simulink model "gm_IP_Core_SS_Switch_and_PWM"  (R2023a)
settings: Solver=VariableStepAuto  StartTime=0.0  StopTime=0.0004  RelTol=1e-3
undefined symbols (not defined in the file or in its folder): f_FPGA_clk, T_FPGA_clk
libraries: hdlsllib x9, simulink x2
(part 3 of 3)

== system gm_IP_Core_SS_Switch_and_PWM/PWM_and_Switching_Signal_Control1/GenPWM/Triangle shift2 ==
  note: Shifts triangle_in signal, if:
      | -direction of triangle_in is down
      | -user input demands a shift smaller than 1/2 of the period
  note: Shifts triangle_in signal, if:
      | -direction of triangle_in is up
      | -user input demands a shift smaller than 1/2 of the period
  note: Shifts triangle_in signal, if:
      | -direction of triangle_in is up
      | -user input demands a shift larger than 1/2 of the period
  note: Shifts triangle_in signal, if:
      | -direction of triangle_in is down
      | -user input demands a shift larger than 1/2 of the period
  note: Detects, if the triangle_wave is increasing or decreasing
  note: modifies triangle_in signal,
      | if the user demands a shift larger than 1/2 period
  triangle_in : Inport
  triangle_shift : Inport  Port=2
  0 : Constant  Value=0  OutDataTypeStr=boolean  SampleTime=T_FPGA_clk
  Data Type Conversion : DataTypeConversion  OutDataTypeStr=fixdt(1,19,17)  SaturateOnIntegerOverflow=off  RndMeth=Floor
  Data Type Conversion1 : DataTypeConversion  OutDataTypeStr=fixdt(1,20,17)  SaturateOnIntegerOverflow=off  RndMeth=Floor
  Delay1 : Delay  DelayLength=1
  Delay2 : Delay  DelayLength=1
  Gain : Gain  Gain=2  OutDataTypeStr=fixdt(1,20,17)
  Gain1 : Gain  Gain=2  OutDataTypeStr=fixdt(1,20,17)
  Relational Operator1 : RelationalOperator  Operator=<=  OutDataTypeStr=boolean  InputSameDT=off
  Relational Operator7 : RelationalOperator  OutDataTypeStr=boolean  InputSameDT=off
  Subsystem : Subsystem
  Subsystem1 : Subsystem
  Subsystem2 : Subsystem
  Subsystem3 : Subsystem
  Sum10 : Sum  Inputs=|-+  OutDataTypeStr=fixdt(1,20,17)
  or : Switch  Criteria=u2 > Threshold  SaturateOnIntegerOverflow=off  InputSameDT=off
  standardized peak of triangle : Constant  OutDataTypeStr=fixdt(0,21,17)  SampleTime=T_FPGA_clk
  sw1 : Switch  Criteria=u2 > Threshold  OutDataTypeStr=fixdt(1,18,16)  SaturateOnIntegerOverflow=off  InputSameDT=off
  sw2 : Switch  Criteria=u2 > Threshold  SaturateOnIntegerOverflow=off  InputSameDT=off
  sw3 : Switch  Criteria=u2 > Threshold  SaturateOnIntegerOverflow=off  InputSameDT=off
  sw4 : Switch  Criteria=u2 > Threshold  Threshold=1  OutDataTypeStr=fixdt(1,20,17)  SaturateOnIntegerOverflow=off  InputSameDT=off
  triangle_sig : Outport  VectorParamsAs1DForOutWhenUnconnected=off
  wires:
  Subsystem3/1(shifted triangle_in signal) -> sw2/3
  Subsystem2/2(enable_out) -> sw1/2
  Subsystem2/1(shifted triangle_in signal) -> sw1/1
  Subsystem1/1(shifted triangle_in signal) -> sw3/1
  Subsystem1/2(enable_out) -> sw3/2, or/1, or/2
  Subsystem/2(enable_out) -> or/3
  Subsystem/1(shifted triangle_in signal) -> sw3/3
  0/1 -> Subsystem/1(Zero_input), Subsystem1/5(Zero_input), Subsystem2/4(Zero_input)
  Delay1/1 -> Relational Operator1/2
  Relational Operator1/1 -> Subsystem2/5(direction down), Subsystem/5(direction down)  "direction down"
  triangle_in/1 -> Data Type Conversion1/1
  Data Type Conversion/1 -> Gain/1
  sw2/1 -> sw1/3
  Gain1/1 -> Sum10/1
  triangle_shift/1 -> Data Type Conversion/1
  standardized peak of triangle/1 -> Gain1/1, Subsystem1/1(standardized peak of triangle), Subsystem2/3(standardized peak of triangle)  "standardized peak of triangle"
  sw1/1 -> triangle_sig/1
  Sum10/1 -> sw4/1
  Gain/1 -> sw4/2, sw4/3, Subsystem1/3(converted triangle_shift), Subsystem/2(converted triangle_shift), Sum10/2  "converted triangle_shift"
  sw4/1 -> Subsystem2/2(modified triangle_shift), Subsystem1/4(modified triangle_shift), Subsystem/3(modified triangle_shift), Subsystem3/2(modified triangle_shift)  "modified triangle_shift"
  or/1 -> sw2/2
  Relational Operator7/1 -> Subsystem3/3(direction up), Subsystem1/6(direction up)  "direction up"
  sw3/1 -> sw2/1
  Data Type Conversion1/1 -> Relational Operator7/1, Delay2/1, Delay1/1, Relational Operator1/1, Subsystem1/2(triangle_in), Subsystem/4(triangle_in), Subsystem2/1(triangle_in), Subsystem3/1(triangle_in)  "triangle_in"
  Delay2/1 -> Relational Operator7/2

== system gm_IP_Core_SS_Switch_and_PWM/PWM_and_Switching_Signal_Control/GenPWM/Counter Ctrl/Delay6_controlled ==
  in0 : Inport  OutDataTypeStr=boolean  SampleTime=1e-08
  stateControl : EnablePort  OutDataTypeStr=boolean
  Delay6 : Delay  DelayLength=double(1)  InitialCondition=0  SampleTime=1e-08
  out0 : Outport  OutDataTypeStr=boolean  SampleTime=1e-08
  wires:
  Delay6/1 -> out0/1
  in0/1 -> Delay6/1

== system gm_IP_Core_SS_Switch_and_PWM/PWM_and_Switching_Signal_Control/GenPWM/Counter Ctrl/Delay_controlled ==
  in0 : Inport  OutDataTypeStr=fixdt(0, 25, 26)  SampleTime=1e-08
  stateControl : EnablePort  OutDataTypeStr=boolean
  Delay : Delay  DelayLength=double(1)  InitialCondition=0  SampleTime=1e-08
  out0 : Outport  OutDataTypeStr=fixdt(0, 25, 26)  SampleTime=1e-08
  wires:
  Delay/1 -> out0/1
  in0/1 -> Delay/1

== system gm_IP_Core_SS_Switch_and_PWM/PWM_and_Switching_Signal_Control/GenPWM/Triangle shift/Subsystem ==
  Zero_input : Inport  OutDataTypeStr=boolean  PortDimensions=1  SampleTime=1e-08
  converted triangle_shift : Inport  Port=2  OutDataTypeStr=fixdt(1, 20, 17)  PortDimensions=1  SampleTime=1e-08
  modified triangle_shift : Inport  Port=3  OutDataTypeStr=fixdt(1, 20, 17)  PortDimensions=1  SampleTime=1e-08
  triangle_in : Inport  Port=4  OutDataTypeStr=fixdt(1, 20, 17)  PortDimensions=1  SampleTime=1e-08
  direction down : Inport  Port=5  OutDataTypeStr=boolean  PortDimensions=1  SampleTime=1e-08
  Relational Operator11 : RelationalOperator  Operator=<=  OutDataTypeStr=boolean  SampleTime=1e-08  InputSameDT=off
  Sum8 : Sum  Inputs=+-  AccumDataTypeStr=fixdt(1, 21, 17)  OutDataTypeStr=fixdt(1, 21, 17)  SampleTime=1e-08
  Unary Minus : UnaryMinus  SampleTime=1e-08
  and2_1 : Switch  Criteria=u2 > Threshold  Threshold=double(0)  OutDataTypeStr=boolean  SampleTime=1e-08  SaturateOnIntegerOverflow=off  InputSameDT=off
  and2_2 : Switch  Criteria=u2 > Threshold  Threshold=double(0)  OutDataTypeStr=boolean  SampleTime=1e-08  SaturateOnIntegerOverflow=off  InputSameDT=off
  shifted triangle_in signal : Outport  SampleTime=1e-08
  enable_out : Outport  Port=2  SampleTime=1e-08
  wires:
  Relational Operator11/1 -> and2_1/2
  Sum8/1 -> shifted triangle_in signal/1
  Unary Minus/1 -> Sum8/1, Relational Operator11/2
  and2_1/1 -> and2_2/1
  and2_2/1 -> enable_out/1
  Zero_input/1 -> and2_2/3, and2_1/3
  converted triangle_shift/1 -> and2_1/1
  modified triangle_shift/1 -> Unary Minus/1
  triangle_in/1 -> Sum8/2, Relational Operator11/1
  direction down/1 -> and2_2/2

== system gm_IP_Core_SS_Switch_and_PWM/PWM_and_Switching_Signal_Control/GenPWM/Triangle shift/Subsystem1 ==
  standardized peak of triangle : Inport  OutDataTypeStr=fixdt(0, 21, 17)  PortDimensions=1  SampleTime=1e-08
  triangle_in : Inport  Port=2  OutDataTypeStr=fixdt(1, 20, 17)  PortDimensions=1  SampleTime=1e-08
  converted triangle_shift : Inport  Port=3  OutDataTypeStr=fixdt(1, 20, 17)  PortDimensions=1  SampleTime=1e-08
  modified triangle_shift : Inport  Port=4  OutDataTypeStr=fixdt(1, 20, 17)  PortDimensions=1  SampleTime=1e-08
  Zero_input : Inport  Port=5  OutDataTypeStr=boolean  PortDimensions=1  SampleTime=1e-08
  direction up : Inport  Port=6  OutDataTypeStr=boolean  PortDimensions=1  SampleTime=1e-08
  Relational Operator2 : RelationalOperator  OutDataTypeStr=boolean  SampleTime=1e-08  InputSameDT=off
  Sum11_stage2 : Sum  AccumDataTypeStr=fixdt(1, 24, 17)  OutDataTypeStr=fixdt(1, 24, 17)  SampleTime=1e-08
  Sum11_stage3 : Sum  Inputs=+-  AccumDataTypeStr=fixdt(1, 24, 17)  OutDataTypeStr=fixdt(1, 21, 17)  SampleTime=1e-08
  Sum6 : Sum  AccumDataTypeStr=fixdt(1, 23, 17)  OutDataTypeStr=fixdt(1, 23, 17)  SampleTime=1e-08
  and1_1 : Switch  Criteria=u2 > Threshold  Threshold=double(0)  OutDataTypeStr=boolean  SampleTime=1e-08  SaturateOnIntegerOverflow=off  InputSameDT=off
  and1_2 : Switch  Criteria=u2 > Threshold  Threshold=double(0)  OutDataTypeStr=boolean  SampleTime=1e-08  SaturateOnIntegerOverflow=off  InputSameDT=off
  shifted triangle_in signal : Outport  SampleTime=1e-08
  enable_out : Outport  Port=2  SampleTime=1e-08
  wires:
  Relational Operator2/1 -> and1_1/2
  Sum11_stage3/1 -> shifted triangle_in signal/1
  Sum6/1 -> Sum11_stage2/2, Relational Operator2/2
  and1_1/1 -> and1_2/1
  and1_2/1 -> enable_out/1
  Sum11_stage2/1 -> Sum11_stage3/1
  standardized peak of triangle/1 -> Sum6/2, Sum11_stage2/1
  triangle_in/1 -> Sum11_stage3/2, Relational Operator2/1
  converted triangle_shift/1 -> and1_1/1
  modified triangle_shift/1 -> Sum6/1
  Zero_input/1 -> and1_2/3, and1_1/3
  direction up/1 -> and1_2/2

== system gm_IP_Core_SS_Switch_and_PWM/PWM_and_Switching_Signal_Control/GenPWM/Triangle shift/Subsystem2 ==
  triangle_in : Inport  OutDataTypeStr=fixdt(1, 20, 17)  PortDimensions=1  SampleTime=1e-08
  modified triangle_shift : Inport  Port=2  OutDataTypeStr=fixdt(1, 20, 17)  PortDimensions=1  SampleTime=1e-08
  standardized peak of triangle : Inport  Port=3  OutDataTypeStr=fixdt(0, 21, 17)  PortDimensions=1  SampleTime=1e-08
  Zero_input : Inport  Port=4  OutDataTypeStr=boolean  PortDimensions=1  SampleTime=1e-08
  direction down : Inport  Port=5  OutDataTypeStr=boolean  PortDimensions=1  SampleTime=1e-08
  Relational Operator9 : RelationalOperator  OutDataTypeStr=boolean  SampleTime=1e-08  InputSameDT=off
  Sum1 : Sum  Inputs=+-  AccumDataTypeStr=fixdt(1, 23, 17)  OutDataTypeStr=fixdt(1, 23, 17)  SampleTime=1e-08
  Sum5_stage2 : Sum  AccumDataTypeStr=fixdt(1, 24, 17)  OutDataTypeStr=fixdt(1, 24, 17)  SampleTime=1e-08
  Sum5_stage3 : Sum  Inputs=+-  AccumDataTypeStr=fixdt(1, 24, 17)  OutDataTypeStr=fixdt(1, 21, 17)  SampleTime=1e-08
  and : Switch  Criteria=u2 > Threshold  Threshold=double(0)  OutDataTypeStr=boolean  SampleTime=1e-08  SaturateOnIntegerOverflow=off  InputSameDT=off
  shifted triangle_in signal : Outport  SampleTime=1e-08
  enable_out : Outport  Port=2  SampleTime=1e-08
  wires:
  Relational Operator9/1 -> and/1
  Sum1/1 -> Sum5_stage2/1, Relational Operator9/2
  Sum5_stage3/1 -> shifted triangle_in signal/1
  and/1 -> enable_out/1
  Sum5_stage2/1 -> Sum5_stage3/1
  triangle_in/1 -> Sum5_stage3/2, Relational Operator9/1
  modified triangle_shift/1 -> Sum1/2
  standardized peak of triangle/1 -> Sum5_stage2/2, Sum1/1
  Zero_input/1 -> and/3
  direction down/1 -> and/2

== system gm_IP_Core_SS_Switch_and_PWM/PWM_and_Switching_Signal_Control/GenPWM/Triangle shift/Subsystem3 ==
  triangle_in : Inport  OutDataTypeStr=fixdt(1, 20, 17)  PortDimensions=1  SampleTime=1e-08
  modified triangle_shift : Inport  Port=2  OutDataTypeStr=fixdt(1, 20, 17)  PortDimensions=1  SampleTime=1e-08
  direction up : Inport  Port=3  OutDataTypeStr=boolean  PortDimensions=1  SampleTime=1e-08
  Relational Operator6 : RelationalOperator  Operator=<=  OutDataTypeStr=boolean  SampleTime=1e-08  InputSameDT=off
  Sum2 : Sum  Inputs=+-  AccumDataTypeStr=fixdt(1, 21, 17)  OutDataTypeStr=fixdt(1, 21, 17)  SampleTime=1e-08
  Sum3 : Sum  Inputs=+-  AccumDataTypeStr=fixdt(1, 21, 17)  OutDataTypeStr=fixdt(1, 21, 17)  SampleTime=1e-08
  Sum4 : Sum  AccumDataTypeStr=fixdt(1, 21, 17)  OutDataTypeStr=fixdt(1, 21, 17)  SampleTime=1e-08
  Switch3 : Switch  Criteria=u2 > Threshold  Threshold=double(0)  OutDataTypeStr=fixdt(1, 21, 17)  SampleTime=1e-08  SaturateOnIntegerOverflow=off  InputSameDT=off
  sw : Switch  Criteria=u2 > Threshold  Threshold=double(0)  OutDataTypeStr=fixdt(1, 21, 17)  SampleTime=1e-08  SaturateOnIntegerOverflow=off  InputSameDT=off
  shifted triangle_in signal : Outport  SampleTime=1e-08
  wires:
  Relational Operator6/1 -> Switch3/2
  Sum2/1 -> Switch3/1
  Sum3/1 -> Switch3/3
  Sum4/1 -> sw/3
  Switch3/1 -> sw/1
  sw/1 -> shifted triangle_in signal/1
  triangle_in/1 -> Sum4/2, Sum3/1, Sum2/2, Relational Operator6/1
  modified triangle_shift/1 -> Sum4/1, Sum3/2, Sum2/1, Relational Operator6/2
  direction up/1 -> sw/2

== system gm_IP_Core_SS_Switch_and_PWM/PWM_and_Switching_Signal_Control/GenPWM/Triangle shift1/Subsystem ==
  Zero_input : Inport  OutDataTypeStr=boolean  PortDimensions=1  SampleTime=1e-08
  converted triangle_shift : Inport  Port=2  OutDataTypeStr=fixdt(1, 20, 17)  PortDimensions=1  SampleTime=1e-08
  modified triangle_shift : Inport  Port=3  OutDataTypeStr=fixdt(1, 20, 17)  PortDimensions=1  SampleTime=1e-08
  triangle_in : Inport  Port=4  OutDataTypeStr=fixdt(1, 20, 17)  PortDimensions=1  SampleTime=1e-08
  direction down : Inport  Port=5  OutDataTypeStr=boolean  PortDimensions=1  SampleTime=1e-08
  Relational Operator11 : RelationalOperator  Operator=<=  OutDataTypeStr=boolean  SampleTime=1e-08  InputSameDT=off
  Sum8 : Sum  Inputs=+-  AccumDataTypeStr=fixdt(1, 21, 17)  OutDataTypeStr=fixdt(1, 21, 17)  SampleTime=1e-08
  Unary Minus : UnaryMinus  SampleTime=1e-08
  and2_1 : Switch  Criteria=u2 > Threshold  Threshold=double(0)  OutDataTypeStr=boolean  SampleTime=1e-08  SaturateOnIntegerOverflow=off  InputSameDT=off
  and2_2 : Switch  Criteria=u2 > Threshold  Threshold=double(0)  OutDataTypeStr=boolean  SampleTime=1e-08  SaturateOnIntegerOverflow=off  InputSameDT=off
  shifted triangle_in signal : Outport  SampleTime=1e-08
  enable_out : Outport  Port=2  SampleTime=1e-08
  wires:
  Relational Operator11/1 -> and2_1/2
  Sum8/1 -> shifted triangle_in signal/1
  Unary Minus/1 -> Sum8/1, Relational Operator11/2
  and2_1/1 -> and2_2/1
  and2_2/1 -> enable_out/1
  Zero_input/1 -> and2_2/3, and2_1/3
  converted triangle_shift/1 -> and2_1/1
  modified triangle_shift/1 -> Unary Minus/1
  triangle_in/1 -> Sum8/2, Relational Operator11/1
  direction down/1 -> and2_2/2

== system gm_IP_Core_SS_Switch_and_PWM/PWM_and_Switching_Signal_Control/GenPWM/Triangle shift1/Subsystem1 ==
  standardized peak of triangle : Inport  OutDataTypeStr=fixdt(0, 21, 17)  PortDimensions=1  SampleTime=1e-08
  triangle_in : Inport  Port=2  OutDataTypeStr=fixdt(1, 20, 17)  PortDimensions=1  SampleTime=1e-08
  converted triangle_shift : Inport  Port=3  OutDataTypeStr=fixdt(1, 20, 17)  PortDimensions=1  SampleTime=1e-08
  modified triangle_shift : Inport  Port=4  OutDataTypeStr=fixdt(1, 20, 17)  PortDimensions=1  SampleTime=1e-08
  Zero_input : Inport  Port=5  OutDataTypeStr=boolean  PortDimensions=1  SampleTime=1e-08
  direction up : Inport  Port=6  OutDataTypeStr=boolean  PortDimensions=1  SampleTime=1e-08
  Relational Operator2 : RelationalOperator  OutDataTypeStr=boolean  SampleTime=1e-08  InputSameDT=off
  Sum11_stage2 : Sum  AccumDataTypeStr=fixdt(1, 24, 17)  OutDataTypeStr=fixdt(1, 24, 17)  SampleTime=1e-08
  Sum11_stage3 : Sum  Inputs=+-  AccumDataTypeStr=fixdt(1, 24, 17)  OutDataTypeStr=fixdt(1, 21, 17)  SampleTime=1e-08
  Sum6 : Sum  AccumDataTypeStr=fixdt(1, 23, 17)  OutDataTypeStr=fixdt(1, 23, 17)  SampleTime=1e-08
  and1_1 : Switch  Criteria=u2 > Threshold  Threshold=double(0)  OutDataTypeStr=boolean  SampleTime=1e-08  SaturateOnIntegerOverflow=off  InputSameDT=off
  and1_2 : Switch  Criteria=u2 > Threshold  Threshold=double(0)  OutDataTypeStr=boolean  SampleTime=1e-08  SaturateOnIntegerOverflow=off  InputSameDT=off
  shifted triangle_in signal : Outport  SampleTime=1e-08
  enable_out : Outport  Port=2  SampleTime=1e-08
  wires:
  Relational Operator2/1 -> and1_1/2
  Sum11_stage3/1 -> shifted triangle_in signal/1
  Sum6/1 -> Sum11_stage2/2, Relational Operator2/2
  and1_1/1 -> and1_2/1
  and1_2/1 -> enable_out/1
  Sum11_stage2/1 -> Sum11_stage3/1
  standardized peak of triangle/1 -> Sum6/2, Sum11_stage2/1
  triangle_in/1 -> Sum11_stage3/2, Relational Operator2/1
  converted triangle_shift/1 -> and1_1/1
  modified triangle_shift/1 -> Sum6/1
  Zero_input/1 -> and1_2/3, and1_1/3
  direction up/1 -> and1_2/2

== system gm_IP_Core_SS_Switch_and_PWM/PWM_and_Switching_Signal_Control/GenPWM/Triangle shift1/Subsystem2 ==
  triangle_in : Inport  OutDataTypeStr=fixdt(1, 20, 17)  PortDimensions=1  SampleTime=1e-08
  modified triangle_shift : Inport  Port=2  OutDataTypeStr=fixdt(1, 20, 17)  PortDimensions=1  SampleTime=1e-08
  standardized peak of triangle : Inport  Port=3  OutDataTypeStr=fixdt(0, 21, 17)  PortDimensions=1  SampleTime=1e-08
  Zero_input : Inport  Port=4  OutDataTypeStr=boolean  PortDimensions=1  SampleTime=1e-08
  direction down : Inport  Port=5  OutDataTypeStr=boolean  PortDimensions=1  SampleTime=1e-08
  Relational Operator9 : RelationalOperator  OutDataTypeStr=boolean  SampleTime=1e-08  InputSameDT=off
  Sum1 : Sum  Inputs=+-  AccumDataTypeStr=fixdt(1, 23, 17)  OutDataTypeStr=fixdt(1, 23, 17)  SampleTime=1e-08
  Sum5_stage2 : Sum  AccumDataTypeStr=fixdt(1, 24, 17)  OutDataTypeStr=fixdt(1, 24, 17)  SampleTime=1e-08
  Sum5_stage3 : Sum  Inputs=+-  AccumDataTypeStr=fixdt(1, 24, 17)  OutDataTypeStr=fixdt(1, 21, 17)  SampleTime=1e-08
  and : Switch  Criteria=u2 > Threshold  Threshold=double(0)  OutDataTypeStr=boolean  SampleTime=1e-08  SaturateOnIntegerOverflow=off  InputSameDT=off
  shifted triangle_in signal : Outport  SampleTime=1e-08
  enable_out : Outport  Port=2  SampleTime=1e-08
  wires:
  Relational Operator9/1 -> and/1
  Sum1/1 -> Sum5_stage2/1, Relational Operator9/2
  Sum5_stage3/1 -> shifted triangle_in signal/1
  and/1 -> enable_out/1
  Sum5_stage2/1 -> Sum5_stage3/1
  triangle_in/1 -> Sum5_stage3/2, Relational Operator9/1
  modified triangle_shift/1 -> Sum1/2
  standardized peak of triangle/1 -> Sum5_stage2/2, Sum1/1
  Zero_input/1 -> and/3
  direction down/1 -> and/2

== system gm_IP_Core_SS_Switch_and_PWM/PWM_and_Switching_Signal_Control/GenPWM/Triangle shift1/Subsystem3 ==
  triangle_in : Inport  OutDataTypeStr=fixdt(1, 20, 17)  PortDimensions=1  SampleTime=1e-08
  modified triangle_shift : Inport  Port=2  OutDataTypeStr=fixdt(1, 20, 17)  PortDimensions=1  SampleTime=1e-08
  direction up : Inport  Port=3  OutDataTypeStr=boolean  PortDimensions=1  SampleTime=1e-08
  Relational Operator6 : RelationalOperator  Operator=<=  OutDataTypeStr=boolean  SampleTime=1e-08  InputSameDT=off
  Sum2 : Sum  Inputs=+-  AccumDataTypeStr=fixdt(1, 21, 17)  OutDataTypeStr=fixdt(1, 21, 17)  SampleTime=1e-08
  Sum3 : Sum  Inputs=+-  AccumDataTypeStr=fixdt(1, 21, 17)  OutDataTypeStr=fixdt(1, 21, 17)  SampleTime=1e-08
  Sum4 : Sum  AccumDataTypeStr=fixdt(1, 21, 17)  OutDataTypeStr=fixdt(1, 21, 17)  SampleTime=1e-08
  Switch3 : Switch  Criteria=u2 > Threshold  Threshold=double(0)  OutDataTypeStr=fixdt(1, 21, 17)  SampleTime=1e-08  SaturateOnIntegerOverflow=off  InputSameDT=off
  sw : Switch  Criteria=u2 > Threshold  Threshold=double(0)  OutDataTypeStr=fixdt(1, 21, 17)  SampleTime=1e-08  SaturateOnIntegerOverflow=off  InputSameDT=off
  shifted triangle_in signal : Outport  SampleTime=1e-08
  wires:
  Relational Operator6/1 -> Switch3/2
  Sum2/1 -> Switch3/1
  Sum3/1 -> Switch3/3
  Sum4/1 -> sw/3
  Switch3/1 -> sw/1
  sw/1 -> shifted triangle_in signal/1
  triangle_in/1 -> Sum4/2, Sum3/1, Sum2/2, Relational Operator6/1
  modified triangle_shift/1 -> Sum4/1, Sum3/2, Sum2/1, Relational Operator6/2
  direction up/1 -> sw/2

== system gm_IP_Core_SS_Switch_and_PWM/PWM_and_Switching_Signal_Control/GenPWM/Triangle shift2/Subsystem ==
  Zero_input : Inport  OutDataTypeStr=boolean  PortDimensions=1  SampleTime=1e-08
  converted triangle_shift : Inport  Port=2  OutDataTypeStr=fixdt(1, 20, 17)  PortDimensions=1  SampleTime=1e-08
  modified triangle_shift : Inport  Port=3  OutDataTypeStr=fixdt(1, 20, 17)  PortDimensions=1  SampleTime=1e-08
  triangle_in : Inport  Port=4  OutDataTypeStr=fixdt(1, 20, 17)  PortDimensions=1  SampleTime=1e-08
  direction down : Inport  Port=5  OutDataTypeStr=boolean  PortDimensions=1  SampleTime=1e-08
  Relational Operator11 : RelationalOperator  Operator=<=  OutDataTypeStr=boolean  SampleTime=1e-08  InputSameDT=off
  Sum8 : Sum  Inputs=+-  AccumDataTypeStr=fixdt(1, 21, 17)  OutDataTypeStr=fixdt(1, 21, 17)  SampleTime=1e-08
  Unary Minus : UnaryMinus  SampleTime=1e-08
  and2_1 : Switch  Criteria=u2 > Threshold  Threshold=double(0)  OutDataTypeStr=boolean  SampleTime=1e-08  SaturateOnIntegerOverflow=off  InputSameDT=off
  and2_2 : Switch  Criteria=u2 > Threshold  Threshold=double(0)  OutDataTypeStr=boolean  SampleTime=1e-08  SaturateOnIntegerOverflow=off  InputSameDT=off
  shifted triangle_in signal : Outport  SampleTime=1e-08
  enable_out : Outport  Port=2  SampleTime=1e-08
  wires:
  Relational Operator11/1 -> and2_1/2
  Sum8/1 -> shifted triangle_in signal/1
  Unary Minus/1 -> Sum8/1, Relational Operator11/2
  and2_1/1 -> and2_2/1
  and2_2/1 -> enable_out/1
  Zero_input/1 -> and2_2/3, and2_1/3
  converted triangle_shift/1 -> and2_1/1
  modified triangle_shift/1 -> Unary Minus/1
  triangle_in/1 -> Sum8/2, Relational Operator11/1
  direction down/1 -> and2_2/2

== system gm_IP_Core_SS_Switch_and_PWM/PWM_and_Switching_Signal_Control/GenPWM/Triangle shift2/Subsystem1 ==
  standardized peak of triangle : Inport  OutDataTypeStr=fixdt(0, 21, 17)  PortDimensions=1  SampleTime=1e-08
  triangle_in : Inport  Port=2  OutDataTypeStr=fixdt(1, 20, 17)  PortDimensions=1  SampleTime=1e-08
  converted triangle_shift : Inport  Port=3  OutDataTypeStr=fixdt(1, 20, 17)  PortDimensions=1  SampleTime=1e-08
  modified triangle_shift : Inport  Port=4  OutDataTypeStr=fixdt(1, 20, 17)  PortDimensions=1  SampleTime=1e-08
  Zero_input : Inport  Port=5  OutDataTypeStr=boolean  PortDimensions=1  SampleTime=1e-08
  direction up : Inport  Port=6  OutDataTypeStr=boolean  PortDimensions=1  SampleTime=1e-08
  Relational Operator2 : RelationalOperator  OutDataTypeStr=boolean  SampleTime=1e-08  InputSameDT=off
  Sum11_stage2 : Sum  AccumDataTypeStr=fixdt(1, 24, 17)  OutDataTypeStr=fixdt(1, 24, 17)  SampleTime=1e-08
  Sum11_stage3 : Sum  Inputs=+-  AccumDataTypeStr=fixdt(1, 24, 17)  OutDataTypeStr=fixdt(1, 21, 17)  SampleTime=1e-08
  Sum6 : Sum  AccumDataTypeStr=fixdt(1, 23, 17)  OutDataTypeStr=fixdt(1, 23, 17)  SampleTime=1e-08
  and1_1 : Switch  Criteria=u2 > Threshold  Threshold=double(0)  OutDataTypeStr=boolean  SampleTime=1e-08  SaturateOnIntegerOverflow=off  InputSameDT=off
  and1_2 : Switch  Criteria=u2 > Threshold  Threshold=double(0)  OutDataTypeStr=boolean  SampleTime=1e-08  SaturateOnIntegerOverflow=off  InputSameDT=off
  shifted triangle_in signal : Outport  SampleTime=1e-08
  enable_out : Outport  Port=2  SampleTime=1e-08
  wires:
  Relational Operator2/1 -> and1_1/2
  Sum11_stage3/1 -> shifted triangle_in signal/1
  Sum6/1 -> Sum11_stage2/2, Relational Operator2/2
  and1_1/1 -> and1_2/1
  and1_2/1 -> enable_out/1
  Sum11_stage2/1 -> Sum11_stage3/1
  standardized peak of triangle/1 -> Sum6/2, Sum11_stage2/1
  triangle_in/1 -> Sum11_stage3/2, Relational Operator2/1
  converted triangle_shift/1 -> and1_1/1
  modified triangle_shift/1 -> Sum6/1
  Zero_input/1 -> and1_2/3, and1_1/3
  direction up/1 -> and1_2/2

== system gm_IP_Core_SS_Switch_and_PWM/PWM_and_Switching_Signal_Control/GenPWM/Triangle shift2/Subsystem2 ==
  triangle_in : Inport  OutDataTypeStr=fixdt(1, 20, 17)  PortDimensions=1  SampleTime=1e-08
  modified triangle_shift : Inport  Port=2  OutDataTypeStr=fixdt(1, 20, 17)  PortDimensions=1  SampleTime=1e-08
  standardized peak of triangle : Inport  Port=3  OutDataTypeStr=fixdt(0, 21, 17)  PortDimensions=1  SampleTime=1e-08
  Zero_input : Inport  Port=4  OutDataTypeStr=boolean  PortDimensions=1  SampleTime=1e-08
  direction down : Inport  Port=5  OutDataTypeStr=boolean  PortDimensions=1  SampleTime=1e-08
  Relational Operator9 : RelationalOperator  OutDataTypeStr=boolean  SampleTime=1e-08  InputSameDT=off
  Sum1 : Sum  Inputs=+-  AccumDataTypeStr=fixdt(1, 23, 17)  OutDataTypeStr=fixdt(1, 23, 17)  SampleTime=1e-08
  Sum5_stage2 : Sum  AccumDataTypeStr=fixdt(1, 24, 17)  OutDataTypeStr=fixdt(1, 24, 17)  SampleTime=1e-08
  Sum5_stage3 : Sum  Inputs=+-  AccumDataTypeStr=fixdt(1, 24, 17)  OutDataTypeStr=fixdt(1, 21, 17)  SampleTime=1e-08
  and : Switch  Criteria=u2 > Threshold  Threshold=double(0)  OutDataTypeStr=boolean  SampleTime=1e-08  SaturateOnIntegerOverflow=off  InputSameDT=off
  shifted triangle_in signal : Outport  SampleTime=1e-08
  enable_out : Outport  Port=2  SampleTime=1e-08
  wires:
  Relational Operator9/1 -> and/1
  Sum1/1 -> Sum5_stage2/1, Relational Operator9/2
  Sum5_stage3/1 -> shifted triangle_in signal/1
  and/1 -> enable_out/1
  Sum5_stage2/1 -> Sum5_stage3/1
  triangle_in/1 -> Sum5_stage3/2, Relational Operator9/1
  modified triangle_shift/1 -> Sum1/2
  standardized peak of triangle/1 -> Sum5_stage2/2, Sum1/1
  Zero_input/1 -> and/3
  direction down/1 -> and/2

== system gm_IP_Core_SS_Switch_and_PWM/PWM_and_Switching_Signal_Control/GenPWM/Triangle shift2/Subsystem3 ==
  triangle_in : Inport  OutDataTypeStr=fixdt(1, 20, 17)  PortDimensions=1  SampleTime=1e-08
  modified triangle_shift : Inport  Port=2  OutDataTypeStr=fixdt(1, 20, 17)  PortDimensions=1  SampleTime=1e-08
  direction up : Inport  Port=3  OutDataTypeStr=boolean  PortDimensions=1  SampleTime=1e-08
  Relational Operator6 : RelationalOperator  Operator=<=  OutDataTypeStr=boolean  SampleTime=1e-08  InputSameDT=off
  Sum2 : Sum  Inputs=+-  AccumDataTypeStr=fixdt(1, 21, 17)  OutDataTypeStr=fixdt(1, 21, 17)  SampleTime=1e-08
  Sum3 : Sum  Inputs=+-  AccumDataTypeStr=fixdt(1, 21, 17)  OutDataTypeStr=fixdt(1, 21, 17)  SampleTime=1e-08
  Sum4 : Sum  AccumDataTypeStr=fixdt(1, 21, 17)  OutDataTypeStr=fixdt(1, 21, 17)  SampleTime=1e-08
  Switch3 : Switch  Criteria=u2 > Threshold  Threshold=double(0)  OutDataTypeStr=fixdt(1, 21, 17)  SampleTime=1e-08  SaturateOnIntegerOverflow=off  InputSameDT=off
  sw : Switch  Criteria=u2 > Threshold  Threshold=double(0)  OutDataTypeStr=fixdt(1, 21, 17)  SampleTime=1e-08  SaturateOnIntegerOverflow=off  InputSameDT=off
  shifted triangle_in signal : Outport  SampleTime=1e-08
  wires:
  Relational Operator6/1 -> Switch3/2
  Sum2/1 -> Switch3/1
  Sum3/1 -> Switch3/3
  Sum4/1 -> sw/3
  Switch3/1 -> sw/1
  sw/1 -> shifted triangle_in signal/1
  triangle_in/1 -> Sum4/2, Sum3/1, Sum2/2, Relational Operator6/1
  modified triangle_shift/1 -> Sum4/1, Sum3/2, Sum2/1, Relational Operator6/2
  direction up/1 -> sw/2

== system gm_IP_Core_SS_Switch_and_PWM/PWM_and_Switching_Signal_Control1/GenPWM/Triangle shift/Subsystem ==
  note: AND block replaced with
      | switches for better performance
  Zero_input : Inport
  converted triangle_shift : Inport  Port=2
  modified triangle_shift : Inport  Port=3
  triangle_in : Inport  Port=4
  direction down : Inport  Port=5
  Relational Operator11 : RelationalOperator  Operator=<=  OutDataTypeStr=boolean  InputSameDT=off
  Sum8 : Sum  Inputs=|-+
  Unary Minus : UnaryMinus
  and2_1 : Switch  Criteria=u2 > Threshold  SaturateOnIntegerOverflow=off  InputSameDT=off
  and2_2 : Switch  Criteria=u2 > Threshold  SaturateOnIntegerOverflow=off  InputSameDT=off
  shifted triangle_in signal : Outport
  enable_out : Outport  Port=2
  wires:
  modified triangle_shift/1 -> Unary Minus/1
  and2_2/1 -> enable_out/1
  converted triangle_shift/1 -> and2_1/1
  triangle_in/1 -> Relational Operator11/1, Sum8/1
  Unary Minus/1 -> Relational Operator11/2, Sum8/2
  Sum8/1 -> shifted triangle_in signal/1
  and2_1/1 -> and2_2/1
  Relational Operator11/1 -> and2_1/2
  Zero_input/1 -> and2_2/3, and2_1/3
  direction down/1 -> and2_2/2

== system gm_IP_Core_SS_Switch_and_PWM/PWM_and_Switching_Signal_Control1/GenPWM/Triangle shift/Subsystem1 ==
  note: AND block replaced with
      | switches for better performance
  note: AND block replaced with
      | switches for better performance
  standardized peak of triangle : Inport
  triangle_in : Inport  Port=2
  converted triangle_shift : Inport  Port=3
  modified triangle_shift : Inport  Port=4
  Zero_input : Inport  Port=5
  direction up : Inport  Port=6
  Relational Operator2 : RelationalOperator  OutDataTypeStr=boolean  InputSameDT=off
  Sum11 : Sum  Inputs=++-  OutDataTypeStr=fixdt(1,21,17)
  Sum6 : Sum  Inputs=++|
  and1_1 : Switch  Criteria=u2 > Threshold  SaturateOnIntegerOverflow=off  InputSameDT=off
  and1_2 : Switch  Criteria=u2 > Threshold  SaturateOnIntegerOverflow=off  InputSameDT=off
  shifted triangle_in signal : Outport
  enable_out : Outport  Port=2
  wires:
  modified triangle_shift/1 -> Sum6/1
  triangle_in/1 -> Sum11/3, Relational Operator2/1
  direction up/1 -> and1_2/2
  converted triangle_shift/1 -> and1_1/1
  and1_2/1 -> enable_out/1
  standardized peak of triangle/1 -> Sum11/1, Sum6/2
  Zero_input/1 -> and1_1/3, and1_2/3
  Relational Operator2/1 -> and1_1/2
  and1_1/1 -> and1_2/1
  Sum6/1 -> Sum11/2, Relational Operator2/2
  Sum11/1 -> shifted triangle_in signal/1

== system gm_IP_Core_SS_Switch_and_PWM/PWM_and_Switching_Signal_Control1/GenPWM/Triangle shift/Subsystem2 ==
  triangle_in : Inport
  modified triangle_shift : Inport  Port=2
  standardized peak of triangle : Inport  Port=3
  Zero_input : Inport  Port=4
  direction down : Inport  Port=5
  Relational Operator9 : RelationalOperator  OutDataTypeStr=boolean  InputSameDT=off
  Sum1 : Sum  Inputs=|-+
  Sum5 : Sum  Inputs=++-  OutDataTypeStr=fixdt(1,21,17)
  and : Switch  Criteria=u2 > Threshold  SaturateOnIntegerOverflow=off  InputSameDT=off
  shifted triangle_in signal : Outport
  enable_out : Outport  Port=2
  wires:
  modified triangle_shift/1 -> Sum1/1
  Sum5/1 -> shifted triangle_in signal/1
  triangle_in/1 -> Sum5/3, Relational Operator9/1
  and/1 -> enable_out/1
  direction down/1 -> and/2
  Relational Operator9/1 -> and/1
  Sum1/1 -> Sum5/1, Relational Operator9/2
  Zero_input/1 -> and/3
  standardized peak of triangle/1 -> Sum5/2, Sum1/2

== system gm_IP_Core_SS_Switch_and_PWM/PWM_and_Switching_Signal_Control1/GenPWM/Triangle shift/Subsystem3 ==
  triangle_in : Inport
  modified triangle_shift : Inport  Port=2
  direction up : Inport  Port=3
  Relational Operator6 : RelationalOperator  Operator=<=  OutDataTypeStr=boolean  InputSameDT=off
  Sum2 : Sum  Inputs=|-+
  Sum3 : Sum  Inputs=|+-
  Sum4 : Sum  Inputs=|++
  Switch3 : Switch  Criteria=u2 > Threshold  SaturateOnIntegerOverflow=off  InputSameDT=off
  sw : Switch  Criteria=u2 > Threshold  SaturateOnIntegerOverflow=off  InputSameDT=off
  shifted triangle_in signal : Outport
  wires:
  triangle_in/1 -> Sum4/2, Sum2/1, Sum3/1, Relational Operator6/1
  direction up/1 -> sw/2
  Relational Operator6/1 -> Switch3/2
  sw/1 -> shifted triangle_in signal/1
  Sum2/1 -> Switch3/1
  Sum3/1 -> Switch3/3
  Switch3/1 -> sw/1
  modified triangle_shift/1 -> Relational Operator6/2, Sum2/2, Sum3/2, Sum4/1
  Sum4/1 -> sw/3

== system gm_IP_Core_SS_Switch_and_PWM/PWM_and_Switching_Signal_Control1/GenPWM/Triangle shift1/Subsystem ==
  note: AND block replaced with
      | switches for better performance
  Zero_input : Inport
  converted triangle_shift : Inport  Port=2
  modified triangle_shift : Inport  Port=3
  triangle_in : Inport  Port=4
  direction down : Inport  Port=5
  Relational Operator11 : RelationalOperator  Operator=<=  OutDataTypeStr=boolean  InputSameDT=off
  Sum8 : Sum  Inputs=|-+
  Unary Minus : UnaryMinus
  and2_1 : Switch  Criteria=u2 > Threshold  SaturateOnIntegerOverflow=off  InputSameDT=off
  and2_2 : Switch  Criteria=u2 > Threshold  SaturateOnIntegerOverflow=off  InputSameDT=off
  shifted triangle_in signal : Outport
  enable_out : Outport  Port=2
  wires:
  modified triangle_shift/1 -> Unary Minus/1
  and2_2/1 -> enable_out/1
  converted triangle_shift/1 -> and2_1/1
  triangle_in/1 -> Relational Operator11/1, Sum8/1
  Unary Minus/1 -> Relational Operator11/2, Sum8/2
  Sum8/1 -> shifted triangle_in signal/1
  and2_1/1 -> and2_2/1
  Relational Operator11/1 -> and2_1/2
  Zero_input/1 -> and2_2/3, and2_1/3
  direction down/1 -> and2_2/2

== system gm_IP_Core_SS_Switch_and_PWM/PWM_and_Switching_Signal_Control1/GenPWM/Triangle shift1/Subsystem1 ==
  note: AND block replaced with
      | switches for better performance
  note: AND block replaced with
      | switches for better performance
  standardized peak of triangle : Inport
  triangle_in : Inport  Port=2
  converted triangle_shift : Inport  Port=3
  modified triangle_shift : Inport  Port=4
  Zero_input : Inport  Port=5
  direction up : Inport  Port=6
  Relational Operator2 : RelationalOperator  OutDataTypeStr=boolean  InputSameDT=off
  Sum11 : Sum  Inputs=++-  OutDataTypeStr=fixdt(1,21,17)
  Sum6 : Sum  Inputs=++|
  and1_1 : Switch  Criteria=u2 > Threshold  SaturateOnIntegerOverflow=off  InputSameDT=off
  and1_2 : Switch  Criteria=u2 > Threshold  SaturateOnIntegerOverflow=off  InputSameDT=off
  shifted triangle_in signal : Outport
  enable_out : Outport  Port=2
  wires:
  modified triangle_shift/1 -> Sum6/1
  triangle_in/1 -> Sum11/3, Relational Operator2/1
  direction up/1 -> and1_2/2
  converted triangle_shift/1 -> and1_1/1
  and1_2/1 -> enable_out/1
  standardized peak of triangle/1 -> Sum11/1, Sum6/2
  Zero_input/1 -> and1_1/3, and1_2/3
  Relational Operator2/1 -> and1_1/2
  and1_1/1 -> and1_2/1
  Sum6/1 -> Sum11/2, Relational Operator2/2
  Sum11/1 -> shifted triangle_in signal/1

== system gm_IP_Core_SS_Switch_and_PWM/PWM_and_Switching_Signal_Control1/GenPWM/Triangle shift1/Subsystem2 ==
  triangle_in : Inport
  modified triangle_shift : Inport  Port=2
  standardized peak of triangle : Inport  Port=3
  Zero_input : Inport  Port=4
  direction down : Inport  Port=5
  Relational Operator9 : RelationalOperator  OutDataTypeStr=boolean  InputSameDT=off
  Sum1 : Sum  Inputs=|-+
  Sum5 : Sum  Inputs=++-  OutDataTypeStr=fixdt(1,21,17)
  and : Switch  Criteria=u2 > Threshold  SaturateOnIntegerOverflow=off  InputSameDT=off
  shifted triangle_in signal : Outport
  enable_out : Outport  Port=2
  wires:
  modified triangle_shift/1 -> Sum1/1
  Sum5/1 -> shifted triangle_in signal/1
  triangle_in/1 -> Sum5/3, Relational Operator9/1
  and/1 -> enable_out/1
  direction down/1 -> and/2
  Relational Operator9/1 -> and/1
  Sum1/1 -> Sum5/1, Relational Operator9/2
  Zero_input/1 -> and/3
  standardized peak of triangle/1 -> Sum5/2, Sum1/2

== system gm_IP_Core_SS_Switch_and_PWM/PWM_and_Switching_Signal_Control1/GenPWM/Triangle shift1/Subsystem3 ==
  triangle_in : Inport
  modified triangle_shift : Inport  Port=2
  direction up : Inport  Port=3
  Relational Operator6 : RelationalOperator  Operator=<=  OutDataTypeStr=boolean  InputSameDT=off
  Sum2 : Sum  Inputs=|-+
  Sum3 : Sum  Inputs=|+-
  Sum4 : Sum  Inputs=|++
  Switch3 : Switch  Criteria=u2 > Threshold  SaturateOnIntegerOverflow=off  InputSameDT=off
  sw : Switch  Criteria=u2 > Threshold  SaturateOnIntegerOverflow=off  InputSameDT=off
  shifted triangle_in signal : Outport
  wires:
  triangle_in/1 -> Sum4/2, Sum2/1, Sum3/1, Relational Operator6/1
  direction up/1 -> sw/2
  Relational Operator6/1 -> Switch3/2
  sw/1 -> shifted triangle_in signal/1
  Sum2/1 -> Switch3/1
  Sum3/1 -> Switch3/3
  Switch3/1 -> sw/1
  modified triangle_shift/1 -> Relational Operator6/2, Sum2/2, Sum3/2, Sum4/1
  Sum4/1 -> sw/3

== system gm_IP_Core_SS_Switch_and_PWM/PWM_and_Switching_Signal_Control1/GenPWM/Triangle shift2/Subsystem ==
  note: AND block replaced with
      | switches for better performance
  Zero_input : Inport
  converted triangle_shift : Inport  Port=2
  modified triangle_shift : Inport  Port=3
  triangle_in : Inport  Port=4
  direction down : Inport  Port=5
  Relational Operator11 : RelationalOperator  Operator=<=  OutDataTypeStr=boolean  InputSameDT=off
  Sum8 : Sum  Inputs=|-+
  Unary Minus : UnaryMinus
  and2_1 : Switch  Criteria=u2 > Threshold  SaturateOnIntegerOverflow=off  InputSameDT=off
  and2_2 : Switch  Criteria=u2 > Threshold  SaturateOnIntegerOverflow=off  InputSameDT=off
  shifted triangle_in signal : Outport
  enable_out : Outport  Port=2
  wires:
  modified triangle_shift/1 -> Unary Minus/1
  and2_2/1 -> enable_out/1
  converted triangle_shift/1 -> and2_1/1
  triangle_in/1 -> Relational Operator11/1, Sum8/1
  Unary Minus/1 -> Relational Operator11/2, Sum8/2
  Sum8/1 -> shifted triangle_in signal/1
  and2_1/1 -> and2_2/1
  Relational Operator11/1 -> and2_1/2
  Zero_input/1 -> and2_2/3, and2_1/3
  direction down/1 -> and2_2/2

== system gm_IP_Core_SS_Switch_and_PWM/PWM_and_Switching_Signal_Control1/GenPWM/Triangle shift2/Subsystem1 ==
  note: AND block replaced with
      | switches for better performance
  note: AND block replaced with
      | switches for better performance
  standardized peak of triangle : Inport
  triangle_in : Inport  Port=2
  converted triangle_shift : Inport  Port=3
  modified triangle_shift : Inport  Port=4
  Zero_input : Inport  Port=5
  direction up : Inport  Port=6
  Relational Operator2 : RelationalOperator  OutDataTypeStr=boolean  InputSameDT=off
  Sum11 : Sum  Inputs=++-  OutDataTypeStr=fixdt(1,21,17)
  Sum6 : Sum  Inputs=++|
  and1_1 : Switch  Criteria=u2 > Threshold  SaturateOnIntegerOverflow=off  InputSameDT=off
  and1_2 : Switch  Criteria=u2 > Threshold  SaturateOnIntegerOverflow=off  InputSameDT=off
  shifted triangle_in signal : Outport
  enable_out : Outport  Port=2
  wires:
  modified triangle_shift/1 -> Sum6/1
  triangle_in/1 -> Sum11/3, Relational Operator2/1
  direction up/1 -> and1_2/2
  converted triangle_shift/1 -> and1_1/1
  and1_2/1 -> enable_out/1
  standardized peak of triangle/1 -> Sum11/1, Sum6/2
  Zero_input/1 -> and1_1/3, and1_2/3
  Relational Operator2/1 -> and1_1/2
  and1_1/1 -> and1_2/1
  Sum6/1 -> Sum11/2, Relational Operator2/2
  Sum11/1 -> shifted triangle_in signal/1

== system gm_IP_Core_SS_Switch_and_PWM/PWM_and_Switching_Signal_Control1/GenPWM/Triangle shift2/Subsystem2 ==
  triangle_in : Inport
  modified triangle_shift : Inport  Port=2
  standardized peak of triangle : Inport  Port=3
  Zero_input : Inport  Port=4
  direction down : Inport  Port=5
  Relational Operator9 : RelationalOperator  OutDataTypeStr=boolean  InputSameDT=off
  Sum1 : Sum  Inputs=|-+
  Sum5 : Sum  Inputs=++-  OutDataTypeStr=fixdt(1,21,17)
  and : Switch  Criteria=u2 > Threshold  SaturateOnIntegerOverflow=off  InputSameDT=off
  shifted triangle_in signal : Outport
  enable_out : Outport  Port=2
  wires:
  modified triangle_shift/1 -> Sum1/1
  Sum5/1 -> shifted triangle_in signal/1
  triangle_in/1 -> Sum5/3, Relational Operator9/1
  and/1 -> enable_out/1
  direction down/1 -> and/2
  Relational Operator9/1 -> and/1
  Sum1/1 -> Sum5/1, Relational Operator9/2
  Zero_input/1 -> and/3
  standardized peak of triangle/1 -> Sum5/2, Sum1/2

== system gm_IP_Core_SS_Switch_and_PWM/PWM_and_Switching_Signal_Control1/GenPWM/Triangle shift2/Subsystem3 ==
  triangle_in : Inport
  modified triangle_shift : Inport  Port=2
  direction up : Inport  Port=3
  Relational Operator6 : RelationalOperator  Operator=<=  OutDataTypeStr=boolean  InputSameDT=off
  Sum2 : Sum  Inputs=|-+
  Sum3 : Sum  Inputs=|+-
  Sum4 : Sum  Inputs=|++
  Switch3 : Switch  Criteria=u2 > Threshold  SaturateOnIntegerOverflow=off  InputSameDT=off
  sw : Switch  Criteria=u2 > Threshold  SaturateOnIntegerOverflow=off  InputSameDT=off
  shifted triangle_in signal : Outport
  wires:
  triangle_in/1 -> Sum4/2, Sum2/1, Sum3/1, Relational Operator6/1
  direction up/1 -> sw/2
  Relational Operator6/1 -> Switch3/2
  sw/1 -> shifted triangle_in signal/1
  Sum2/1 -> Switch3/1
  Sum3/1 -> Switch3/3
  Switch3/1 -> sw/1
  modified triangle_shift/1 -> Relational Operator6/2, Sum2/2, Sum3/2, Sum4/1
  Sum4/1 -> sw/3
